simulink model "CalcPhat"  (Simulink 6.5)
settings: Solver=FixedStepDiscrete  StartTime=0.0  StopTime=0.0  RelTol=1e-3
libraries: dspxfrm3 x1
settings Model: Creator=cameraman  LastModifiedBy=cameraman  ExtModeAutoUpdateStatusClock=off
settings OptimizationCC: OptimizeModelRefInitCode=on  LifeSpan=1
settings RTWCC: SystemTargetFile=ert.tlc  TemplateMakefile=ert_default_tmf  Description=Real-Time Workshop Embedded Coder (no auto configuration)  GenerateReport=on  ProcessScript=ert_make_rtw_hook  IncludeHyperlinkInReport=on  LaunchReport=on
settings CodeAppCC: IgnoreCustomStorageClasses=off
settings ERTTargetCC: TargetFcnLib=ansi_tfl_tmw.mat  GenFloatMathFcnCalls=ANSI_C  GenerateSampleERTMain=on  InlinedParameterPlacement=NonHierarchical  ERTCustomFileTemplate=example_file_process.tlc

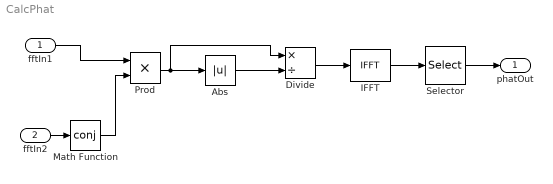
== system CalcPhat ==
  fftIn1 : Inport  PortDimensions=[8192 1]  DataType=single
      settings: SignalType=complex
  fftIn2 : Inport  Port=2  PortDimensions=[8192 1]  DataType=single
      settings: SignalType=complex
  Abs : Abs
  Divide : Product  Inputs=*/  OutScaling=2^-10
  IFFT : dspxfrm3/IFFT  DialogController=dspDDGCreate  DialogControllerArgs=DataTag0  CompMethod=Table lookup  TableOpt=Speed  BitRevOrder=off  cs_in=on  SkipNorm=off  mode=Complex  roundingMode=Floor  overflowMode=off
  Math Function : Math  Operator=conj  SaturateOnIntegerOverflow=on
  Prod : Product  RndMeth=Zero
  Selector : Selector  InputType=Vector  ElementSrc=Internal  Elements=[7992:8192 1:200]  RowSrc=Internal  Rows=1  ColumnSrc=Internal  Columns=1  IndexIsStartValue=off
  phatOut : Outport  DataType=single
  wires:
  IFFT/1 -> Selector/1
  Selector/1 -> phatOut/1
  Prod/1 -> Abs/1, Divide/1
  Abs/1 -> Divide/2
  Divide/1 -> IFFT/1
  fftIn1/1 -> Prod/1
  fftIn2/1 -> Math Function/1
  Math Function/1 -> Prod/2
